simulink model "F16sim_K_q"  (R2023b)
settings: Solver=ode4  StartTime=0  StopTime=5  FixedStep=0.01  RelTol=1e-3  EnableMultiTasking=on
values from neighbouring files (symbols this model uses):
  fc = 1/2    (= 0.5)    [runsim_K_q.m]
  Kq = 2    [runsim_K_q.m]
undefined symbols (not defined in the file or in its folder): A_lon, B_lon, C, C_lon, CA, D_lon, invCB
settings Model: Creator=keviczky  LastModifiedBy=suvo
settings DataIOCC: Decimation=50  SaveFormat=Array  SignalLoggingSaveFormat=ModelDataLogs  ReturnWorkspaceOutputs=off  SignalLoggingName=sigsOut
settings OptimizationCC: BooleanDataType=off
settings DebuggingCC: SaveWithParameterizedLinksMsg=none  UnderspecifiedInitializationDetection=Classic  MergeDetectMultiDrivingBlocksExec=none  SignalResolutionControl=TryResolveAllWithWarning  MultiTaskDSMMsg=warning  MultiTaskCondExecSysMsg=none  UnconnectedInputMsg=warning  UnconnectedOutputMsg=warning  UnconnectedLineMsg=warning
settings HardwareCC: ProdBitPerPointer=32  ProdBitPerSizeT=32  ProdBitPerPtrDiffT=32  ProdLargestAtomicFloat=None  ProdIntDivRoundTo=Undefined  ProdEndianess=Unspecified  ProdWordSize=32  ProdHWDeviceType=32-bit Generic  TargetUnknown=on
settings ModelReferenceCC: PropagateSignalLabelsOutOfModel=off
settings GRTTargetCC: CombineOutputUpdateFcns=off  GRTInterface=on
settings ConfigComp: CovMetricSettings=dw  CovSaveCumulativeToWorkspaceVar=on  CovSaveSingleToWorkspaceVar=on

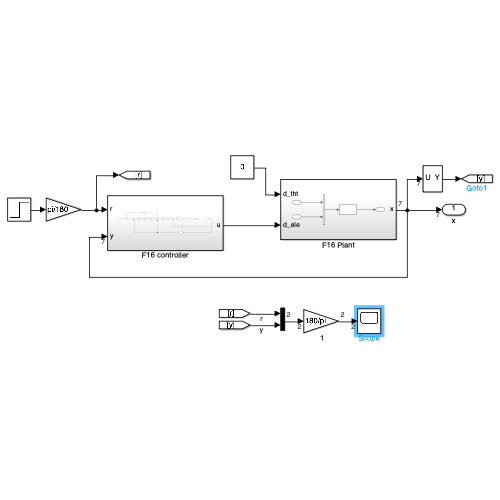
[thumbnail: Simulink's stored preview of the top-level diagram]
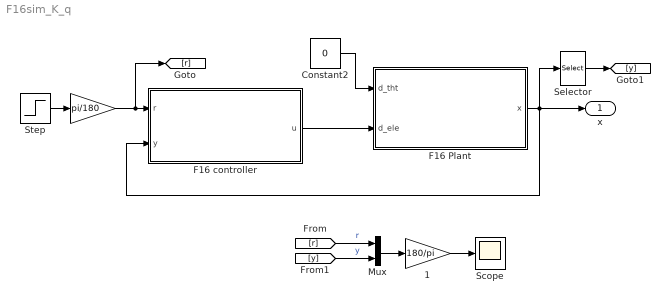
== system F16sim_K_q ==
  " " : Gain  Gain=pi/180
  " 1" : Gain  Gain=180/pi
  Constant2 : Constant  Value=0
  F16 Plant : Subsystem
  F16 controller : Subsystem
  Mux : Mux  Inputs=2
  Scope : Scope
  Selector : Selector  InputPortWidth=7  IndexOptions=Index vector (dialog)  Indices=4  OutputSizes=1
  Step : Step  SampleTime=0
  x : Outport
  wires:
  Constant2/1 -> F16 Plant/1(d_tht)
  F16 Plant/1(x) -> Selector/1, F16 controller/2(y), x/1
  Step/1 -> " "/1
  F16 controller/1(u) -> F16 Plant/2(d_ele)
  [r] -> Mux/1  "r"
  [y] -> Mux/2  "y"
  Mux/1 -> " 1"/1
  Selector/1 -> [y]
  " "/1 -> F16 controller/1(r), [r]
  " 1"/1 -> Scope/1

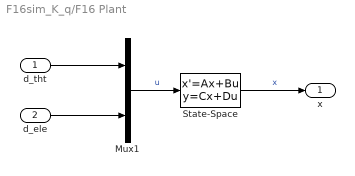
== system F16sim_K_q/F16 Plant ==
  d_tht : Inport
  d_ele : Inport  Port=2
  Mux1 : Mux  Inputs=2
  State-Space : StateSpace  A=A_lon  B=B_lon  C=C_lon  D=D_lon  InitialCondition=0
  x : Outport
  wires:
  d_tht/1 -> Mux1/1
  Mux1/1 -> State-Space/1  "u"
  d_ele/1 -> Mux1/2
  State-Space/1 -> x/1  "x"

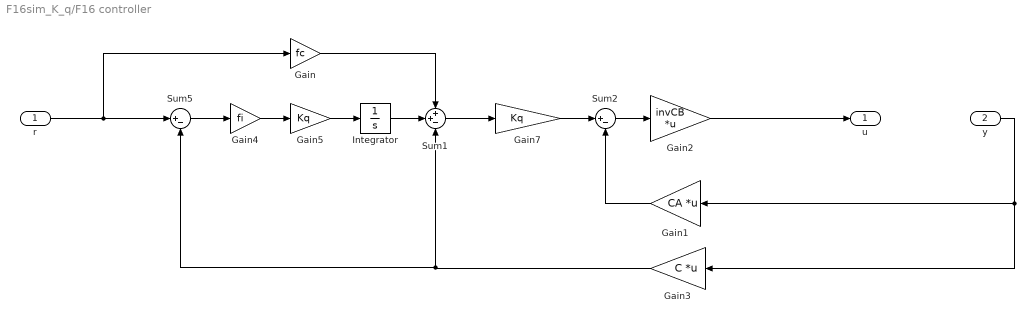
== system F16sim_K_q/F16 controller ==
  r : Inport
  y : Inport  Port=2
  Gain : Gain  Gain=fc
  Gain1 : Gain  Gain=CA  Multiplication=Matrix(K*u)
  Gain2 : Gain  Gain=invCB  Multiplication=Matrix(K*u)
  Gain3 : Gain  Gain=C  Multiplication=Matrix(K*u)
  Gain4 : Gain  Gain=fi
  Gain5 : Gain  Gain=Kq
  Gain7 : Gain  Gain=Kq
  Integrator : Integrator
  Sum1 : Sum  Inputs=++-
  Sum2 : Sum  Inputs=|+-
  Sum5 : Sum  Inputs=|+-
  u : Outport
  wires:
  Gain2/1 -> u/1
  Sum1/1 -> Gain7/1
  r/1 -> Gain/1, Sum5/1
  y/1 -> Gain3/1, Gain1/1
  Gain5/1 -> Integrator/1
  Sum2/1 -> Gain2/1
  Gain1/1 -> Sum2/2
  Gain/1 -> Sum1/1
  Sum5/1 -> Gain4/1
  Gain4/1 -> Gain5/1
  Gain3/1 -> Sum1/3, Sum5/2
  Gain7/1 -> Sum2/1
  Integrator/1 -> Sum1/2
